simulink model "exercise_05_simscape"  (R2022b)
settings: Solver=VariableStepAuto  StartTime=0.0  StopTime=10*2*pi/w  MaxStep=(2*pi/w)*1e-4  MinStep=(2*pi/w)*1e-12  RelTol=1e-3  AbsTol=1e-3
model workspace (MAT data in the model file):
  R = 5
  XC = -10
  XL = 15
  XM = 5
  a = 1
  gm = 0.1
  w = 6.28318530718
libraries: fl_lib x10, nesl_utility x3
settings Model: Creator=paolo  LastModifiedBy=stefa
settings SolverCC: AutoScaleAbsTol=off  AlgebraicLoopSolver=TrustRegion  MaxZcPerStep=1
settings DebuggingCC: UnconnectedInputMsg=warning  UnconnectedOutputMsg=warning  UnconnectedLineMsg=warning  SymbolicDimsDataTypeCodeGenerationDiagnostic=none
settings ModelReferenceCC: EnableRefExpFcnMdlSchedulingChecks=on
settings SFSimCC: CustomCodeUndefinedFunction=UseInterfaceOnly
settings RTWCC: DLArmComputeVersion=19.05
settings SimscapeCC: SimscapeLogType=all  SimscapeLogSimulationStatistics=on  SimscapeLogDataHistory=10000

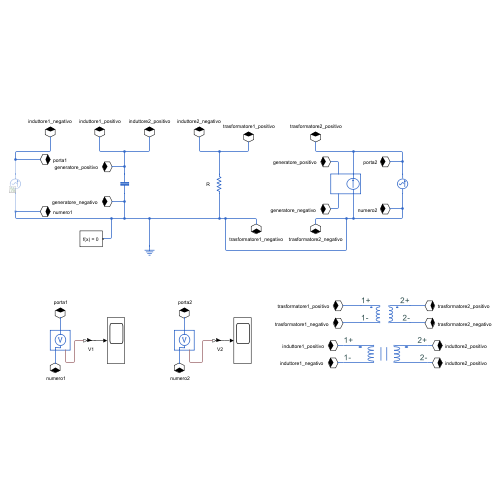
[thumbnail: Simulink's stored preview of the top-level diagram]
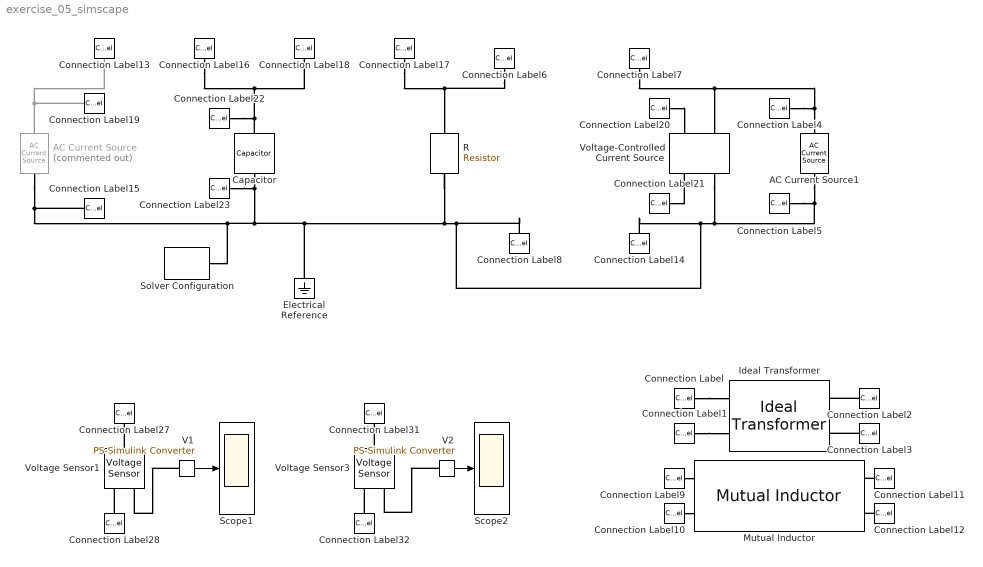
== system exercise_05_simscape ==
  AC Current Source : fl_lib/Electrical/Electrical Sources/AC Current Source  Commented=on  amp=1 A  shift=pi/2 rad  frequency=w/(2*pi) Hz  omega=0 rad/s
      settings: InternalSimscapePortConfiguration="{\"Bottom\":[],\"Left\":[{\"id\":\"p\",\"label\":\"\",\"type\":\"foundation.electrical.electrical\"}],\"Right\":[{\"id\":\"n\",\"label\":\"\",\"type\":\"foundation.electrical.electrical\"}],\"Top\":[]}"
  AC Current Source1 : fl_lib/Electrical/Electrical Sources/AC Current Source  amp=1 A  shift=pi/2 rad  frequency=w/(2*pi) Hz  omega=0 rad/s
      settings: InternalSimscapePortConfiguration="{\"Bottom\":[],\"Left\":[{\"id\":\"p\",\"label\":\"\",\"type\":\"foundation.electrical.electrical\"}],\"Right\":[{\"id\":\"n\",\"label\":\"\",\"type\":\"foundation.electrical.electrical\"}],\"Top\":[]}"
  Capacitor : fl_lib/Electrical/Electrical Elements/Capacitor  c=-1/w*XC F  r=0 Ohm  g=0 1/Ohm  i_specify=off  i_priority=None  i=0 A  i_nominal_specify=off  i_nominal_unit=A  i_nominal_value=1  v_specify=off  v_priority=None  v=0 V  v_nominal_specify=off  v_nominal_unit=V  v_nominal_value=1  vc_specify=off  vc_priority=High  vc=0 V  vc_nominal_specify=off  vc_nominal_unit=V  vc_nominal_value=1
  Connection Label : ConnectionLabel  Label=trasformatore1_positivo
  Connection Label1 : ConnectionLabel  Label=trasformatore1_negativo
  Connection Label10 : ConnectionLabel  Label=induttore1_negativo
  Connection Label11 : ConnectionLabel  Label=induttore2_positivo
  Connection Label12 : ConnectionLabel  Label=induttore2_positivo
  Connection Label13 : ConnectionLabel  Label=induttore1_negativo
  Connection Label14 : ConnectionLabel  Label=trasformatore2_negativo
  Connection Label15 : ConnectionLabel  Label=numero1
  Connection Label16 : ConnectionLabel  Label=induttore1_positivo
  Connection Label17 : ConnectionLabel  Label=induttore2_negativo
  Connection Label18 : ConnectionLabel  Label=induttore2_positivo
  Connection Label19 : ConnectionLabel  Label=porta1
  Connection Label2 : ConnectionLabel  Label=trasformatore2_positivo
  Connection Label20 : ConnectionLabel  Label=generatore_positivo
  Connection Label21 : ConnectionLabel  Label=generatore_negativo
  Connection Label22 : ConnectionLabel  Label=generatore_positivo
  Connection Label23 : ConnectionLabel  Label=generatore_negativo
  Connection Label27 : ConnectionLabel  Label=porta1
  Connection Label28 : ConnectionLabel  Label=numero1
  Connection Label3 : ConnectionLabel  Label=trasformatore2_negativo
  Connection Label31 : ConnectionLabel  Label=porta2
  Connection Label32 : ConnectionLabel  Label=numero2
  Connection Label4 : ConnectionLabel  Label=porta2
  Connection Label5 : ConnectionLabel  Label=numero2
  Connection Label6 : ConnectionLabel  Label=trasformatore1_positivo
  Connection Label7 : ConnectionLabel  Label=trasformatore2_positivo
  Connection Label8 : ConnectionLabel  Label=trasformatore1_negativo
  Connection Label9 : ConnectionLabel  Label=induttore1_positivo
  Electrical Reference : fl_lib/Electrical/Electrical Elements/Electrical Reference
  Ideal Transformer : fl_lib/Electrical/Electrical Elements/Ideal Transformer  n=a  i1_specify=off  i1_priority=None  i1=0 A  i1_nominal_specify=off  i1_nominal_unit=A  i1_nominal_value=1  v1_specify=off  v1_priority=None  v1=0 V  v1_nominal_specify=off  v1_nominal_unit=V  v1_nominal_value=1  i2_specify=off  i2_priority=None  i2=0 A  i2_nominal_specify=off  i2_nominal_unit=A  i2_nominal_value=1  v2_specify=off  v2_priority=None  v2=0 V  v2_nominal_specify=off  v2_nominal_unit=V  v2_nominal_value=1
  Mutual Inductor : fl_lib/Electrical/Electrical Elements/Mutual Inductor  L1=XL/w H  L2=XL/w H  k=XM/XL  i1_specify=off  i1_priority=High  i1=0 A  i1_nominal_specify=off  i1_nominal_unit=A  i1_nominal_value=1  i2_specify=off  i2_priority=High  i2=0 A  i2_nominal_specify=off  i2_nominal_unit=A  i2_nominal_value=1  v1_specify=off  v1_priority=None  v1=0 V  v1_nominal_specify=off  v1_nominal_unit=V  v1_nominal_value=1  v2_specify=off  v2_priority=None  v2=0 V  v2_nominal_specify=off  v2_nominal_unit=V  v2_nominal_value=1
      settings: InternalSimscapePortConfiguration="{\"Bottom\":[],\"Left\":[{\"id\":\"p1\",\"label\":\"1+\",\"type\":\"foundation.electrical.electrical\"},{\"id\":\"n1\",\"label\":\"1-\",\"type\":\"foundation.electrical.electrical\"}],\"Right\":[{\"id\":\"p2\",\"label\":\"2+\",\"type\":\"foundation.electrical.electrical\"},{\"id\":\"n2\",\"label\":\"2-\",\"type\":\"foundation.electrical.electrical\"}],\"Top\":[]}"
  R : fl_lib/Electrical/Electrical Elements/Resistor  R=R Ohm  i_specify=off  i_priority=None  i=0 A  i_nominal_specify=off  i_nominal_unit=A  i_nominal_value=1  v_specify=off  v_priority=None  v=0 V  v_nominal_specify=off  v_nominal_unit=V  v_nominal_value=1
  Scope1 : Scope
  Scope2 : Scope
  Solver Configuration : nesl_utility/Solver Configuration  PhysicalDomain=network_engine_domain  SubClassName=solver  LeftPortType=input  RightPortType=generic  Tones=[]  Harmonics=[]  SimulateNoise=off  Profile=off  UseLocalSampling=off  EnableSwitchedLinearOptims=on  FrequencyDomain=off  UseCCode=off  RelTol=0.001  AbsTol=0.001  MinStep=1e-09  ToWorkspace=off  RevertToSquareIcSolve=off  NumHomotopyIterations=100  PhasorMode=off  PhasorModeNumHarmonics=1  ConsistencySolver=NEWTON_XTOL_AFTER_FTOL  IndexReductionMethod=DerivativeReplacement  DoDC=off  ResidualTolerance=1e-09  ConsistencyTolSource=GLOBAL  ConsistencyAbsTol=0.001  ConsistencyRelTol=0.001  ConsistencyTolFactor=0.001  UseLocalSolver=off  LocalSolverChoice=NE_BACKWARD_EULER_ADVANCER  ResolveIndetEquations=on  FunctionEvalNumThread=1  LocalSolverSampleTime=0.001  DoFixedCost=off  MaxNonlinIter=3  MaxModeIter=2  ComputeImpulses=off  ImpulseIterations=2  LinearAlgebra=auto  LinearAlgebraNumThread=0  EquationFormulation=NE_TIME_EF  DelaysMemoryBudget=1024  AutomaticFiltering=on  FilteringTimeConstant=0.001  PartitionStorageMethod=AS_NEEDED  PartitionMemoryBudget=1024  PartitionMethod=ROBUST
  V1 : nesl_utility/PS-Simulink Converter  PhysicalDomain=network_engine_domain  SubClassName=ps_output  LeftPortType=input  RightPortType=output  PseudoPeriodic=off  Frequencies=[]  VectorFormat=1-D array  Unit=inherit  AffineConversion=off
  V2 : nesl_utility/PS-Simulink Converter  PhysicalDomain=network_engine_domain  SubClassName=ps_output  LeftPortType=input  RightPortType=output  PseudoPeriodic=off  Frequencies=[]  VectorFormat=1-D array  Unit=inherit  AffineConversion=off
  Voltage Sensor1 : fl_lib/Electrical/Electrical Sensors/Voltage Sensor
  Voltage Sensor3 : fl_lib/Electrical/Electrical Sensors/Voltage Sensor
  Voltage-Controlled Current Source : fl_lib/Electrical/Electrical Sources/Voltage-Controlled Current Source  K=gm 1/Ohm  v1_specify=off  v1_priority=None  v1=0 V  v1_nominal_specify=off  v1_nominal_unit=V  v1_nominal_value=1  i2_specify=off  i2_priority=None  i2=0 A  i2_nominal_specify=off  i2_nominal_unit=A  i2_nominal_value=1
      settings: InternalSimscapePortConfiguration="{\"Bottom\":[],\"Left\":[{\"id\":\"p1\",\"label\":\"+\",\"type\":\"foundation.electrical.electrical\"},{\"id\":\"head\",\"label\":\"\",\"type\":\"foundation.electrical.electrical\"}],\"Right\":[{\"id\":\"n1\",\"label\":\"-\",\"type\":\"foundation.electrical.electrical\"},{\"id\":\"tail\",\"label\":\"\",\"type\":\"foundation.electrical.electrical\"}],\"Top\":[]}"
  wires:
  V1/1 -> Scope1/1
  V2/1 -> Scope2/1
  connections:
  Connection Label6/LConn1 -- Connection Label17/LConn1 -- R/LConn1
  Connection Label1/LConn1 -- Ideal Transformer/LConn2
  Connection Label3/LConn1 -- Ideal Transformer/RConn2
  Connection Label2/LConn1 -- Ideal Transformer/RConn1
  Connection Label/LConn1 -- Ideal Transformer/LConn1
  Voltage-Controlled Current Source/RConn2 -- Connection Label14/LConn1 -- Connection Label8/LConn1 -- Electrical Reference/LConn1 -- Connection Label23/LConn1 -- Capacitor/RConn1 -- Connection Label15/LConn1 -- AC Current Source/RConn1 -- Solver Configuration/RConn1 -- R/RConn1 -- AC Current Source1/RConn1 -- Connection Label5/LConn1
  Connection Label9/LConn1 -- Mutual Inductor/LConn1
  Connection Label10/LConn1 -- Mutual Inductor/LConn2
  Connection Label11/LConn1 -- Mutual Inductor/RConn1
  Connection Label12/LConn1 -- Mutual Inductor/RConn2
  AC Current Source/LConn1 -- Connection Label19/LConn1 -- Connection Label13/LConn1
  Capacitor/LConn1 -- Connection Label22/LConn1 -- Connection Label18/LConn1 -- Connection Label16/LConn1
  Connection Label20/LConn1 -- Voltage-Controlled Current Source/LConn1
  Connection Label21/LConn1 -- Voltage-Controlled Current Source/RConn1
  Connection Label7/LConn1 -- AC Current Source1/LConn1 -- Connection Label4/LConn1 -- Voltage-Controlled Current Source/LConn2
  Voltage Sensor3/LConn1 -- Connection Label31/LConn1
  V1/LConn1 -- Voltage Sensor1/RConn1
  Connection Label32/LConn1 -- Voltage Sensor3/RConn2
  Connection Label28/LConn1 -- Voltage Sensor1/RConn2
  V2/LConn1 -- Voltage Sensor3/RConn1
  Voltage Sensor1/LConn1 -- Connection Label27/LConn1
